simulink model "Mixed_Radix_IFFT_Stream_Ex1"  (R2023a)
settings: Solver=VariableStepAuto  StartTime=0.0  StopTime=1  RelTol=1e-3
undefined symbols (not defined in the file): None, Radix, S, vsva2197, xcvc1902
libraries: dspxfrm3 x2, aieUtilities x2, aieDSP x2, dspsrcs4 x1, vmcUtilities x1
settings Model: Creator=sdegala  LastModifiedBy=robg
settings ModelReferenceCC: EnableRefExpFcnMdlSchedulingChecks=on

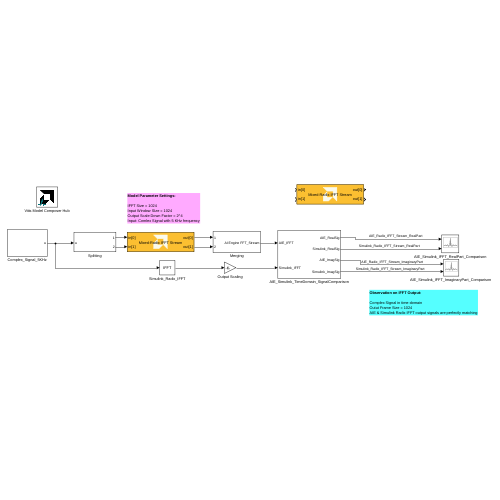
[thumbnail: Simulink's stored preview of the top-level diagram]
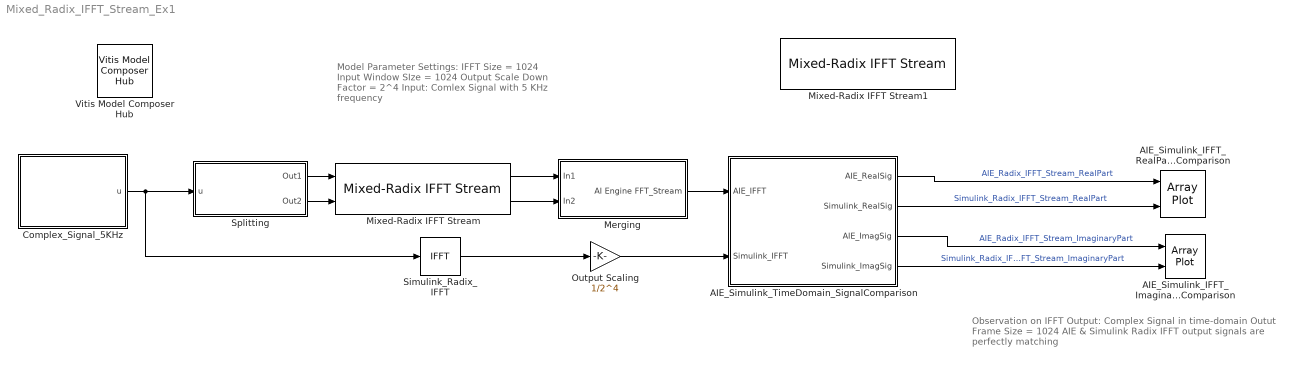
== system Mixed_Radix_IFFT_Stream_Ex1 ==
  note: Observation on IFFT Output:
      |
      | Complex Signal in time-domain
      | Outut Frame Size = 1024
      | AIE & Simulink Radix IFFT output signals are perfectly matching
  note: Model Parameter Settings:
      |
      | IFFT Size = 1024
      | Input Window SIze = 1024
      | Output Scale Down Factor = 2^4
      | Input: Comlex Signal with 5 KHz frequency
  "AIE_Simulink_IFFT_ImaginaryPart_Comparison " : ArrayPlot  NumInputPorts=2  WindowPosition=[2.000000,37.000000,1280.000000,655.000000,]  PlotType=Line  AxesScaling=Manual  YLimits=[-100,100]  ShowLegend=on
  AIE_Simulink_IFFT_RealPart_Comparison : ArrayPlot  NumInputPorts=2  WindowPosition=[5.000000,41.000000,1272.000000,651.000000,]  PlotType=Line  YLimits=[-80,80]  ShowLegend=on
  AIE_Simulink_TimeDomain_SignalComparison : Subsystem
  Complex_Signal_5KHz : Subsystem
  Merging : Subsystem
  Mixed-Radix IFFT Stream : aieDSP/Mixed-Radix IFFT Stream  AIE_VARIANT=1  data_type=cint16  twiddle_type=cint16  point_size=1024  input_window_size=1024  dyn_pt_size=0  casc_length=1  shift_val=4  rnd_mode=Round symmetrical to infinity  sat_mode=0-None  blockJsonConstraints=[]  blockJsonConstraintsInternal=[]  spec=vmc_stream_mixed_radix_ifft.json  SerializedMaskParamNames=[]  SerializedMaskParamValues=[]  SerializedMaskParamVisibilities=[]  block_type=Mixed-Radix IFFT Stream  SerializedMaskParamDataypes=uint|typename|typename|uint|uint|uint|uint|uint|uint|uint  SerializedMaskParamEnumStrArr=0|0|0|0|0|0|0|0|Round to positive infinity,Round to negative infinity,Round symmetrical to infinity,Round symmetrical to zero,Round convergent to even,Round convergent to odd|0-None,1-Asymmetric,3-Symmetric  SerializedMaskParamEnumValArr=0|0|0|0|0|0|0|0|2,3,4,5,6,7|0,1,3  SerializedMaskParamVectorArr=0|0|0|0|0|0|0|0|0|0
  Mixed-Radix IFFT Stream1 : aieDSP/Mixed-Radix IFFT Stream  AIE_VARIANT=1  data_type=cint16  twiddle_type=cint16  point_size=1024  input_window_size=1024  dyn_pt_size=0  casc_length=1  shift_val=4  rnd_mode=Round symmetrical to infinity  sat_mode=0-None  blockJsonConstraints=[]  blockJsonConstraintsInternal=[]  spec=vmc_stream_mixed_radix_ifft.json  SerializedMaskParamNames=[]  SerializedMaskParamValues=[]  SerializedMaskParamVisibilities=[]  block_type=Mixed-Radix IFFT Stream  SerializedMaskParamDataypes=uint|typename|typename|uint|uint|uint|uint|uint|uint|uint  SerializedMaskParamEnumStrArr=0|0|0|0|0|0|0|0|Round to positive infinity,Round to negative infinity,Round symmetrical to infinity,Round symmetrical to zero,Round convergent to even,Round convergent to odd|0-None,1-Asymmetric,3-Symmetric  SerializedMaskParamEnumValArr=0|0|0|0|0|0|0|0|2,3,4,5,6,7|0,1,3  SerializedMaskParamVectorArr=0|0|0|0|0|0|0|0|0|0
  Output Scaling : Gain  Gain=1/2^4
  Simulink_Radix_IFFT : dspxfrm3/IFFT  FFTImplementation=Radix-2  CompMethod=Table lookup  TableOpt=NEW  TableOptActive=Speed  BitRevOrder=off  cs_in=off  Normalize=off  InheritFFTLength=on  FFTLength=64  WrapInput=on  mode=Complex  outSamplingMode=Sample based  roundingMode=Floor  overflowMode=off  firstCoeffDataTypeStr=Inherit: Same word length as input  firstCoeffLastDataTypeStr=Inherit: Same word length as input  prodOutputMode=Binary point scaling  prodOutputWordLength=24  prodOutputFracLength=0  prodOutputDataTypeStr=fixdt(1,24,0)  prodOutputLastDataTypeStr=fixdt(1,24,0)  outputMode=Binary point scaling  outputWordLength=16  outputFracLength=0  outputDataTypeStr=fixdt(1,16,0)  outputMin=[]  outputMax=[]  outputLastDataTypeStr=fixdt(1,16,0)
  Splitting : Subsystem
  Vitis Model Composer Hub : vmcUtilities/Vitis Model Composer Hub  Tag=genX  CodeGeneration=off  StartColumn=1  NumberOfColumns=1  TargetDirectory=./code  exportDesign=off  analyzeDesign=off  validateDesignOnHw=off  ExportType=AI Engines  IpVendor=xilinx.com  IpLibrary=hls  IpVersion=1.0  IpHWLanguage=Verilog  AieCompilerOptions={}  AieSimulatorOptions={}  CreateTestbench=off  TestbenchStackSize=10  RunRtlSim=off  RunCSim=off  RunAieSim=off  AieSimTimeout=50000  RunAieSimProfiling=off  LaunchVitisAnalyzer=off  PlotOutput=off  RunX86Sim=off  X86SimTimeout=10  GenHwImage=off  GenLibadfXo=off  GenHwValidationCode=off  PlatformType=Not Specified  HwSystemType=Baremetal  HwValidationTarget=hw  ProjDevice=xcvc1902-vsva2197-1LP-e-S  ProjDevicePart=xcvc1902-vsva2197-1LP-e-S  AIEType=AIE  SamplePeriod=-1  ClockFrequency=200  DataPathParallelism=1  xilinxfamily=versalaicore  part=xcvc1902  speed=-1LP-e-S  package=vsva2197  directory=./netlist  testbench=off  incr_netlist=off  synthesis_tool=Vivado  clock_wrapper=Clock Enables  dbl_ovrd=According to Block Masks  dcm_input_clock_period=10  sysclk_period=10  simulink_period=1  eval_field=0  LogFileName=''  NThreads=4
  wires:
  AIE_Simulink_TimeDomain_SignalComparison/1(AIE_RealSig) -> AIE_Simulink_IFFT_RealPart_Comparison/1  "AIE_Radix_IFFT_Stream_RealPart"
  AIE_Simulink_TimeDomain_SignalComparison/4(Simulink_ImagSig) -> "AIE_Simulink_IFFT_ImaginaryPart_Comparison "/2  "Simulink_Radix_IFFT_Stream_ImaginaryPart"
  Simulink_Radix_IFFT/1 -> Output Scaling/1
  AIE_Simulink_TimeDomain_SignalComparison/2(Simulink_RealSig) -> AIE_Simulink_IFFT_RealPart_Comparison/2  "Simulink_Radix_IFFT_Stream_RealPart"
  AIE_Simulink_TimeDomain_SignalComparison/3(AIE_ImagSig) -> "AIE_Simulink_IFFT_ImaginaryPart_Comparison "/1  "AIE_Radix_IFFT_Stream_ImaginaryPart"
  Complex_Signal_5KHz/1(u) -> Splitting/1(u), Simulink_Radix_IFFT/1
  Splitting/1(Out1) -> Mixed-Radix IFFT Stream/1
  Splitting/2(Out2) -> Mixed-Radix IFFT Stream/2
  Mixed-Radix IFFT Stream/1 -> Merging/1(In1)
  Mixed-Radix IFFT Stream/2 -> Merging/2(In2)
  Merging/1(AI Engine FFT_Stream) -> AIE_Simulink_TimeDomain_SignalComparison/1(AIE_IFFT)
  Output Scaling/1 -> AIE_Simulink_TimeDomain_SignalComparison/2(Simulink_IFFT)

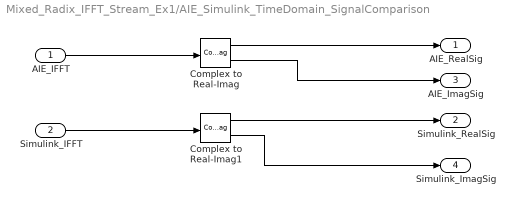
== system Mixed_Radix_IFFT_Stream_Ex1/AIE_Simulink_TimeDomain_SignalComparison ==
  AIE_IFFT : Inport
  Simulink_IFFT : Inport  Port=2
  Complex to Real-Imag : ComplexToRealImag
  Complex to Real-Imag1 : ComplexToRealImag
  AIE_RealSig : Outport
  Simulink_RealSig : Outport  Port=2
  AIE_ImagSig : Outport  Port=3
  Simulink_ImagSig : Outport  Port=4
  wires:
  AIE_IFFT/1 -> Complex to Real-Imag/1
  Complex to Real-Imag/1 -> AIE_RealSig/1
  Complex to Real-Imag1/1 -> Simulink_RealSig/1
  Complex to Real-Imag1/2 -> Simulink_ImagSig/1
  Complex to Real-Imag/2 -> AIE_ImagSig/1
  Simulink_IFFT/1 -> Complex to Real-Imag1/1

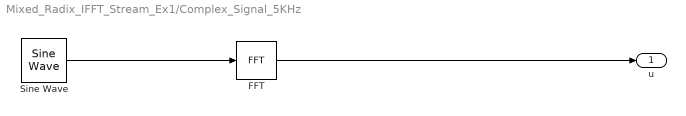
== system Mixed_Radix_IFFT_Stream_Ex1/Complex_Signal_5KHz ==
  FFT : dspxfrm3/FFT  FFTImplementation=Radix-2  CompMethod=Table lookup  TableOpt=NEW  TableOptActive=Speed  BitRevOrder=off  Normalize=off  InheritFFTLength=on  FFTLength=64  WrapInput=on  roundingMode=Floor  overflowMode=off  firstCoeffDataTypeStr=Inherit: Same word length as input  firstCoeffLastDataTypeStr=Inherit: Same word length as input  outputMode=Binary point scaling  outputWordLength=16  outputFracLength=0  outputDataTypeStr=fixdt(1,16,0)  outputMin=[]  outputMax=[]  outputLastDataTypeStr=fixdt(1,16,0)
  Sine Wave : dspsrcs4/Sine Wave  Amplitude=1  Frequency=5e3  Phase=0  SampleMode=Discrete  OutComplex=Complex  CompMethod=Table lookup  TableSize=Speed  SampleTime=1/20e3  SamplesPerFrame=1024  ResetState=Restart at time zero  OutputFrames=off  dataType=Fixed-point  wordLen=16  udDataType=sfix(16)  fracBitsMode=User-defined  numFracBits=14  OutDataTypeStr=fixdt(1,16,14)  LastOutDataTypeStr=fixdt(1,16,14)
  u : Outport
  wires:
  Sine Wave/1 -> FFT/1
  FFT/1 -> u/1

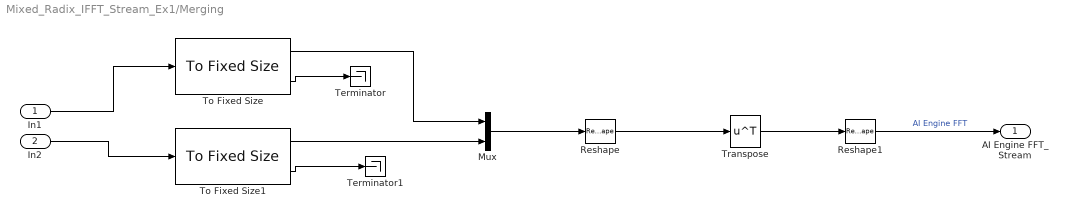
== system Mixed_Radix_IFFT_Stream_Ex1/Merging ==
  In1 : Inport
  In2 : Inport  Port=2
  Mux : Mux  Inputs=2
  Reshape : Reshape  OutputDimensionality=Customize  OutputDimensions=[512, 2]
  Reshape1 : Reshape  OutputDimensions=[1, 10]
  Terminator : Terminator
  Terminator1 : Terminator
  To Fixed Size : aieUtilities/To Fixed Size  Mode=Produce a valid output signal  OutputSize=Inherit: Same as input  CopyMethod=Buffer samples to form output  HasStatusOutput=on
  To Fixed Size1 : aieUtilities/To Fixed Size  Mode=Produce a valid output signal  OutputSize=Inherit: Same as input  CopyMethod=Buffer samples to form output  HasStatusOutput=on
  Transpose : Math  Operator=transpose
  AI Engine FFT_Stream : Outport
  wires:
  Reshape/1 -> Transpose/1
  To Fixed Size1/2 -> Terminator1/1
  To Fixed Size1/1 -> Mux/2
  In2/1 -> To Fixed Size1/1
  To Fixed Size/2 -> Terminator/1
  Transpose/1 -> Reshape1/1
  To Fixed Size/1 -> Mux/1
  Mux/1 -> Reshape/1
  Reshape1/1 -> AI Engine FFT_Stream/1  "AI Engine FFT"
  In1/1 -> To Fixed Size/1

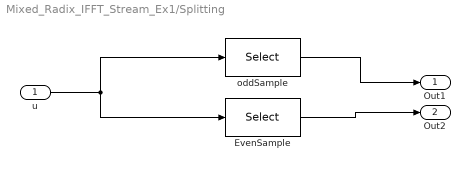
== system Mixed_Radix_IFFT_Stream_Ex1/Splitting ==
  u : Inport
  EvenSample : Selector  InputPortWidth=1024  IndexOptions=Index vector (dialog)  Indices=2:2:1024  OutputSizes=1
  oddSample : Selector  InputPortWidth=1024  IndexOptions=Index vector (dialog)  Indices=1:2:1024  OutputSizes=1
  Out1 : Outport
  Out2 : Outport  Port=2
  wires:
  u/1 -> oddSample/1, EvenSample/1
  EvenSample/1 -> Out2/1
  oddSample/1 -> Out1/1
